simulink model "point_cloud_fusion_node"  (R2016b)
settings: Solver=FixedStepAuto  StartTime=0.0  StopTime=10.0  RelTol=1e-3
model workspace (MAT data in the model file):
  Logfile_Data_Object = [3707764736; 2; 1; 1; 1; 4]
  Logfile_Path = 'C:\Users\takum\MATLAB\Projects\Autoware.Auto\ros2bag\lidars_point_raw\lidars_point_raw_0.db3'
  Logfile_Playback_Duration = nan
  Logfile_Playback_Offset = nan
  SL_ROS_VariableLengthArrays_MaxSizes.CommonInfo.ArrayTruncateAction = 'EmitWarning'
  SL_ROS_VariableLengthArrays_MaxSizes.MsgTypeMap = containers.Map
  SL_ROS_VariableLengthArrays_MaxSizes.MsgTypeMap.serialization.keys = {'sensor_msgs/PointCloud2'}
  SL_ROS_VariableLengthArrays_MaxSizes.MsgTypeMap.serialization.values{1}(1).PropertyName = 'data'
  SL_ROS_VariableLengthArrays_MaxSizes.MsgTypeMap.serialization.values{1}(1).DataType = 'uint8'
  SL_ROS_VariableLengthArrays_MaxSizes.MsgTypeMap.serialization.values{1}(1).MaxLength = 130752
  SL_ROS_VariableLengthArrays_MaxSizes.MsgTypeMap.serialization.values{1}(2).PropertyName = 'fields'
  SL_ROS_VariableLengthArrays_MaxSizes.MsgTypeMap.serialization.values{1}(2).DataType = 'sensor_msgs/PointField'
  SL_ROS_VariableLengthArrays_MaxSizes.MsgTypeMap.serialization.values{1}(2).MaxLength = 16
  SL_ROS_VariableLengthArrays_MaxSizes.MsgTypeMap.serialization.uniformity = 0
  SL_ROS_VariableLengthArrays_MaxSizes.MsgTypeMap.serialization.keyType = 'char'
  SL_ROS_VariableLengthArrays_MaxSizes.MsgTypeMap.serialization.valueType = 'any'
undefined symbols (not defined in the file): data, header, height, row_step, width
libraries: simulink x4
settings Model: Creator=takum  LastModifiedBy=takum
settings DataIOCC: ReturnWorkspaceOutputs=on
settings OptimizationCC: EnhancedBackFolding=on  PassReuseOutputArgsAs=Individual arguments  MaxStackSize=64
settings DebuggingCC: ParameterTunabilityLossMsg=error
settings SFSimCC: SimUseLocalCustomCode=on
settings RTWCC: SystemTargetFile=ert.tlc  HardwareBoard=Robot Operating System 2 (ROS 2)  TLCOptions=-aInlineSetEventsForThisBaseRateFcn=TLC_FALSE -aSuppressMultiTaskScheduler=TLC_FALSE -aRateBasedStepFcn=1  TemplateMakefile=ert_default_tmf  Description=Embedded Coder  RTWUseLocalCustomCode=on  Toolchain=Colcon Tools  TargetLang=C++
settings CodeAppCC: ForceParamTrailComments=on  IgnoreCustomStorageClasses=off  OperatorAnnotations=on  SimulinkDataObjDesc=on  SFDataObjDesc=on  InsertBlockDesc=on
settings ERTTargetCC: MultiwordLength=256  MultiInstanceERTCode=on  CodeInterfacePackaging=C++ class  RootIOFormat=Structure reference

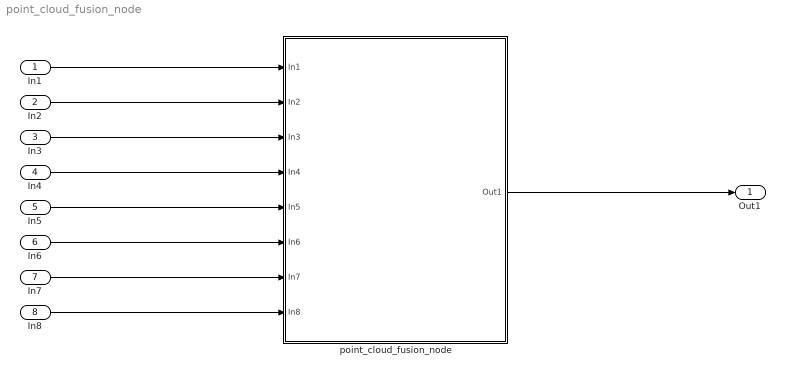
== system point_cloud_fusion_node ==
  In1 : Inport  OutDataTypeStr=Bus: SL_Bus_sensor_msgs_PointCloud2
  In2 : Inport  Port=2  OutDataTypeStr=Bus: SL_Bus_sensor_msgs_PointCloud2
  In3 : Inport  Port=3  OutDataTypeStr=Bus: SL_Bus_sensor_msgs_PointCloud2
  In4 : Inport  Port=4  OutDataTypeStr=Bus: SL_Bus_sensor_msgs_PointCloud2
  In5 : Inport  Port=5  OutDataTypeStr=Bus: SL_Bus_sensor_msgs_PointCloud2
  In6 : Inport  Port=6  OutDataTypeStr=Bus: SL_Bus_sensor_msgs_PointCloud2
  In7 : Inport  Port=7  OutDataTypeStr=Bus: SL_Bus_sensor_msgs_PointCloud2
  In8 : Inport  Port=8  OutDataTypeStr=Bus: SL_Bus_sensor_msgs_PointCloud2
  point_cloud_fusion_node : Subsystem  TreatAsAtomicUnit=on
  Out1 : Outport  OutDataTypeStr=Bus: SL_Bus_sensor_msgs_PointCloud2
  wires:
  point_cloud_fusion_node/1(Out1) -> Out1/1
  In1/1 -> point_cloud_fusion_node/1(In1)
  In2/1 -> point_cloud_fusion_node/2(In2)
  In3/1 -> point_cloud_fusion_node/3(In3)
  In4/1 -> point_cloud_fusion_node/4(In4)
  In5/1 -> point_cloud_fusion_node/5(In5)
  In6/1 -> point_cloud_fusion_node/6(In6)
  In7/1 -> point_cloud_fusion_node/7(In7)
  In8/1 -> point_cloud_fusion_node/8(In8)

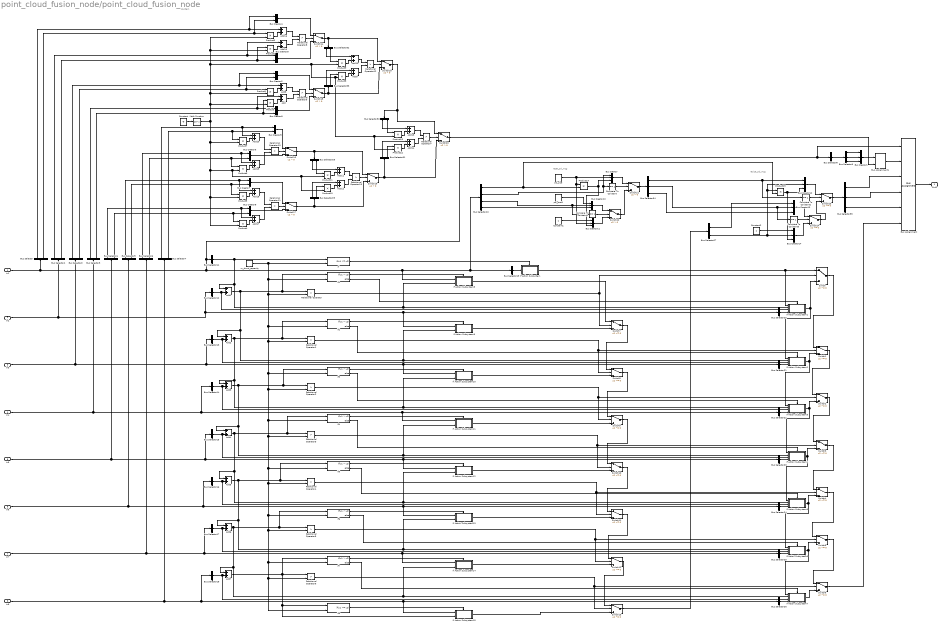
== system point_cloud_fusion_node/point_cloud_fusion_node ==
  note: Subsystem
  note: reset_pcl_msg
  note: resize_pcl_msg
  In1 : Inport
  In2 : Inport  Port=2
  In3 : Inport  Port=3
  In4 : Inport  Port=4
  In5 : Inport  Port=5
  In6 : Inport  Port=6
  In7 : Inport  Port=7
  In8 : Inport  Port=8
  Add{,1..20} (21 alike) : Sum
  Bus Assignment : BusAssignment  AssignedSignals=header,height,width,row_step,data
  Bus Assignment1 : BusAssignment  AssignedSignals=stamp
  Bus Creator{,1,10..14} (7 alike) : BusCreator  Inputs=3
  Bus Creator{2..9} (8 alike) : BusCreator  Inputs=2
  Bus Selector{,1..7} (8 alike) : BusSelector  OutputSignals=header.stamp.sec,header.stamp.nanosec
  Bus Selector10 : BusSelector  OutputSignals=point_step,height,width,row_step
  Bus Selector{11..18} (8 alike) : BusSelector  OutputSignals=width
  Bus Selector{19..26} (8 alike) : BusSelector  OutputSignals=data
  Bus Selector27 : BusSelector  OutputSignals=height,width
  Bus Selector{28..33} (6 alike) : BusSelector  OutputSignals=sec,nanosec
  Bus Selector34 : BusSelector  OutputSignals=height,width,row_step
  Bus Selector35 : BusSelector  OutputSignals=height,width,row_step
  Bus Selector8 : BusSelector  OutputSignals=header
  Bus Selector9 : BusSelector  OutputSignals=stamp,frame_id,frame_id_SL_Info
  Compare To Constant{,1..3} (4 alike) : simulink/Logic and Bit Operations/Compare To Constant  relop===  const=1  OutDataTypeStr=boolean
  Constant : Constant  Value=-9
  Constant1 : Constant
  Constant2 : Constant
  If : If  NumInputs=2  IfExpression=u1 <= u2  ShowElse=off
  If Action Subsystem : Subsystem  TreatAsAtomicUnit=on
  If Action Subsystem1 : Subsystem  TreatAsAtomicUnit=on
  If Action Subsystem10 : Subsystem  TreatAsAtomicUnit=on
  If Action Subsystem11 : Subsystem  TreatAsAtomicUnit=on
  If Action Subsystem12 : Subsystem  TreatAsAtomicUnit=on
  If Action Subsystem13 : Subsystem  TreatAsAtomicUnit=on
  If Action Subsystem14 : Subsystem  TreatAsAtomicUnit=on
  If Action Subsystem15 : Subsystem  TreatAsAtomicUnit=on
  If Action Subsystem2 : Subsystem  TreatAsAtomicUnit=on
  If Action Subsystem3 : Subsystem  TreatAsAtomicUnit=on
  If Action Subsystem4 : Subsystem  TreatAsAtomicUnit=on
  If Action Subsystem5 : Subsystem  TreatAsAtomicUnit=on
  If Action Subsystem6 : Subsystem  TreatAsAtomicUnit=on
  If Action Subsystem7 : Subsystem  TreatAsAtomicUnit=on
  If Action Subsystem8 : Subsystem  TreatAsAtomicUnit=on
  If Action Subsystem9 : Subsystem  TreatAsAtomicUnit=on
  If{1..7} (7 alike) : If  NumInputs=2  IfExpression=u1 > u2
  If8 : If  NumInputs=2  IfExpression=u1 <= u2  ShowElse=off
  Math Function : Math  Operator=10^u  SaturateOnIntegerOverflow=on
  Product{,1..15} (16 alike) : Product
  Relational Operator{,1..13} (14 alike) : RelationalOperator  Operator=>  OutDataTypeStr=boolean  RndMeth=Simplest
  Switch{,1..13,23..24} (16 alike) : Switch  Criteria=u2 ~= 0
  Switch{14..22} (9 alike) : Switch  Criteria=u2 > Threshold
  m_cloud_capacity : Constant  Value=55000  OutDataTypeStr=uint32
  pcl_size : Constant  Value=55000
  pcl_size1 : Constant  Value=55000
  Out1 : Outport
  wires:
  In1/1 -> Bus Selector/1, Bus Selector11/1, Bus Assignment/1, Bus Selector8/1, Bus Selector19/1, Bus Selector10/1, If Action Subsystem8/1(In1)
  Relational Operator12/1 -> Switch18/2
  If4/1 -> If Action Subsystem11/Action
  Compare To Constant1/1 -> Switch22/2
  Bus Creator/1 -> Switch21/1
  If Action Subsystem9/1(Out1) -> Switch7/3
  Bus Selector1/1 -> Add15/1, Bus Creator3/1  "<sec>"
  If Action Subsystem1/1(msgs) -> Switch/3, If Action Subsystem2/1(In1)
  In8/1 -> Bus Selector7/1, If Action Subsystem15/1(In1), Bus Selector26/1, Bus Selector18/1
  Relational Operator11/1 -> Switch17/2
  Bus Selector34/3 -> Bus Creator13/3  "<row_step>"
  If5/1 -> If Action Subsystem12/Action
  If7/2 -> If Action Subsystem7/Action
  Bus Selector1/2 -> Product2/1, Bus Creator3/2  "<nanosec>"
  Add15/1 -> Relational Operator8/2
  Add20/1 -> Relational Operator10/1
  Bus Selector33/1 -> Add9/1  "<sec>"
  Switch10/1 -> Switch11/1
  Compare To Constant/1 -> Switch21/2
  If Action Subsystem2/1(msgs) -> If Action Subsystem3/1(In1), Switch1/3
  Bus Selector10/1 -> Product15/2, Product14/2  "<point_step>"
  Bus Selector19/1 -> If Action Subsystem/1(pc_in)  "<data>"
  In3/1 -> Bus Selector2/1, Bus Selector13/1, Bus Selector21/1, If Action Subsystem10/1(In1)
  Product4/1 -> Add17/2
  Switch21/1 -> Bus Selector34/1
  Bus Selector6/1 -> Add19/1, Bus Creator6/1  "<sec>"
  Constant2/1 -> Bus Creator14/1  "height"
  Relational Operator6/1 -> Switch13/2, Switch6/2
  Product3/1 -> Add16/2
  If Action Subsystem7/1(msgs) -> Switch6/3
  Product14/1 -> Bus Creator11/3, Bus Creator/3  "row_step"
  Switch9/1 -> Switch10/1
  If1/1 -> If Action Subsystem8/Action
  Compare To Constant3/1 -> Switch24/2
  Bus Assignment/1 -> Out1/1
  Product15/1 -> Bus Creator12/3, Bus Creator14/3  "row_step"
  Bus Selector14/1 -> If Action Subsystem3/3(In3), Add3/2  "<width>"
  Bus Creator10/1 -> Switch22/1
  Compare To Constant2/1 -> Switch23/2
  Switch23/1 -> Bus Selector35/1
  If Action Subsystem12/1(Out1) -> Switch10/3
  Product2/1 -> Add15/2
  Bus Selector2/1 -> Bus Creator2/1, Add8/1  "<sec>"
  Bus Creator6/1 -> Switch16/3
  Relational Operator13/1 -> Switch19/2
  Bus Selector7/1 -> Add20/1, Bus Creator5/1  "<sec>"
  Relational Operator7/1 -> Switch20/2
  If3/1 -> If Action Subsystem10/Action
  Relational Operator8/1 -> Switch14/2
  Bus Creator12/1 -> Switch23/1
  Bus Selector21/1 -> If Action Subsystem2/4(pc_in)  "<data>"
  Switch4/1 -> Switch5/1
  Bus Selector24/1 -> If Action Subsystem5/4(pc_in)  "<data>"
  Switch2/1 -> Switch3/1
  Bus Selector27/2 -> Bus Creator12/2, Product15/1, Bus Creator14/2  "<width>"
  Bus Selector31/2 -> Product12/1  "<nanosec>"
  Bus Selector35/1 -> Bus Assignment/3  "<height>"
  If Action Subsystem3/1(msgs) -> If Action Subsystem4/1(In1), Switch2/3
  Switch14/1 -> Switch18/1, Bus Selector32/1
  Bus Selector23/1 -> If Action Subsystem4/4(pc_in)  "<data>"
  If6/2 -> If Action Subsystem6/Action
  If Action Subsystem11/1(Out1) -> Switch9/3
  Product6/1 -> Add19/2
  Product7/1 -> Add20/2
  Add3/1 -> If3/1, Relational Operator2/1, Add4/1, If Action Subsystem4/2(<width>), If Action Subsystem11/2(In2)
  Add2/1 -> If2/1, Relational Operator1/1, If Action Subsystem10/2(In2), If Action Subsystem3/2(<width>), Add3/1
  Bus Assignment1/1 -> Bus Assignment/2
  Relational Operator9/1 -> Switch15/2
  Switch3/1 -> Switch4/1
  If4/2 -> If Action Subsystem4/Action
  Add13/1 -> Relational Operator7/1
  Bus Selector30/2 -> Product13/1  "<nanosec>"
  Bus Selector28/1 -> Add11/1  "<sec>"
  Relational Operator10/1 -> Switch16/2
  Product/1 -> Add/2
  Bus Selector10/3 -> Compare To Constant1/1, Bus Creator10/2  "<width>"
  Bus Selector7/2 -> Bus Creator5/2, Product7/1  "<nanosec>"
  Bus Creator13/1 -> Switch24/1
  Bus Selector34/1 -> Compare To Constant2/1, Bus Creator12/1  "<height>"
  Switch/1 -> Switch1/1
  If2/2 -> If Action Subsystem2/Action
  If3/2 -> If Action Subsystem3/Action
  Bus Selector10/4 -> Bus Creator10/3  "<row_step>"
  Add16/1 -> Relational Operator8/1
  Add1/1 -> If Action Subsystem9/2(In2), If Action Subsystem2/2(<width>), Add2/1, Relational Operator/1, If1/1
  Bus Selector9/1 -> Bus Creator1/1  "<stamp>"
  Bus Selector5/2 -> Bus Creator7/2, Product5/1  "<nanosec>"
  In6/1 -> Bus Selector5/1, Bus Selector24/1, If Action Subsystem13/1(In1), Bus Selector16/1
  Add/1 -> Relational Operator9/2
  Switch12/1 -> Switch13/1
  Math Function/1 -> Product4/2, Product5/2, Product10/2, Product11/2, Product6/2, Product7/2, Product2/2, Product3/2, Product13/2, Product12/2, Product8/2, Product9/2, Product1/2, Product/2
  If Action Subsystem/1(msgs) -> If Action Subsystem1/1(In1), Switch/1
  Bus Selector35/2 -> Bus Assignment/4  "<width>"
  Bus Selector10/2 -> Bus Creator/1, Compare To Constant/1  "<height>"
  Bus Selector18/1 -> If Action Subsystem7/3(In3), Add7/2  "<width>"
  pcl_size/1 -> Bus Creator/2, Bus Creator11/2, Product14/1  "width"
  Bus Selector29/1 -> Add12/1  "<sec>"
  Bus Selector6/2 -> Bus Creator6/2, Product6/1  "<nanosec>"
  Bus Creator11/1 -> Switch22/3
  Bus Selector9/2 -> Bus Creator1/2  "<frame_id>"
  Product8/1 -> Add9/2
  Bus Selector25/1 -> If Action Subsystem6/4(pc_in)  "<data>"
  If Action Subsystem15/1(Out1) -> Switch13/3
  If Action Subsystem13/1(Out1) -> Switch11/3
  Switch22/1 -> Switch21/3
  Switch17/1 -> Switch19/3, Bus Selector29/1
  Bus Selector34/2 -> Compare To Constant3/1, Bus Creator13/2  "<width>"
  Bus Creator9/1 -> Switch15/3
  If Action Subsystem8/1(Out1) -> Switch7/1
  Relational Operator3/1 -> Switch10/2, Switch3/2
  Switch18/1 -> Bus Selector30/1, Switch20/1
  Add18/1 -> Relational Operator11/1
  In7/1 -> Bus Selector6/1, If Action Subsystem14/1(In1), Bus Selector25/1, Bus Selector17/1
  Relational Operator2/1 -> Switch2/2, Switch9/2
  Add14/1 -> Relational Operator7/2
  Product5/1 -> Add18/2
  Add17/1 -> Relational Operator11/2
  Bus Selector17/1 -> If Action Subsystem6/3(In3), Add6/2  "<width>"
  If1/2 -> If Action Subsystem1/Action
  Product12/1 -> Add14/2
  Switch19/1 -> Bus Selector31/1, Switch20/3
  If2/1 -> If Action Subsystem9/Action
  Bus Creator2/1 -> Switch15/1
  Add8/1 -> Relational Operator9/1
  Add9/1 -> Relational Operator12/2
  Bus Creator14/1 -> Switch24/3
  If8/1 -> If Action Subsystem15/Action
  In4/1 -> Bus Selector3/1, If Action Subsystem11/1(In1), Bus Selector22/1, Bus Selector14/1
  Bus Creator1/1 -> Bus Assignment1/1
  Product10/1 -> Add12/2
  Add6/1 -> If Action Subsystem14/2(In2), If Action Subsystem7/2(<width>), Add7/1, If6/1, Relational Operator5/1
  Switch1/1 -> Switch2/1
  Switch6/1 -> Bus Assignment/6  "data"
  Add5/1 -> If5/1, Relational Operator4/1, If Action Subsystem13/2(In2), If Action Subsystem6/2(<width>), Add6/1
  If Action Subsystem4/1(msgs) -> If Action Subsystem5/1(In1), Switch3/3
  Product1/1 -> Add8/2
  Add11/1 -> Relational Operator13/1
  Constant1/1 -> Bus Creator11/1  "height"
  If Action Subsystem10/1(Out1) -> Switch8/3
  If Action Subsystem5/1(msgs) -> If Action Subsystem6/1(In1), Switch4/3
  If7/1 -> If Action Subsystem14/Action
  Bus Selector12/1 -> If Action Subsystem1/3(In3), Add1/2  "<width>"
  Add12/1 -> Relational Operator13/2
  If5/2 -> If Action Subsystem5/Action
  Constant/1 -> Math Function/1
  Switch24/1 -> Switch23/3
  Bus Creator8/1 -> Switch17/3
  Bus Selector15/1 -> If Action Subsystem4/3(In3), Add4/2  "<width>"
  Bus Creator7/1 -> Switch17/1
  Switch5/1 -> Switch6/1
  Switch20/1 -> Bus Assignment1/2  "header.stamp"
  Bus Selector9/3 -> Bus Creator1/3  "<frame_id_SL_Info>"
  Bus Selector33/2 -> Product8/1  "<nanosec>"
  Bus Selector/1 -> Add16/1, Bus Creator4/1  "<sec>"
  Bus Selector20/1 -> If Action Subsystem1/4(pc_in)  "<data>"
  Relational Operator5/1 -> Switch12/2, Switch5/2
  Bus Selector29/2 -> Product10/1  "<nanosec>"
  Product13/1 -> Add13/2
  Bus Creator5/1 -> Switch16/1
  Bus Selector8/1 -> Bus Selector9/1  "<header>"
  Bus Selector22/1 -> If Action Subsystem3/4(pc_in)  "<data>"
  m_cloud_capacity/1 -> Relational Operator3/2, Relational Operator4/2, If8/2, Relational Operator6/2, If7/2, Relational Operator5/2, If6/2, If5/2, If4/2, Relational Operator2/2, If3/2, Relational Operator1/2, If2/2, Relational Operator/2, If1/2, If/2
  Add10/1 -> Relational Operator12/1
  Add7/1 -> If8/1, If Action Subsystem15/2(In2), If7/1, Relational Operator6/1
  Bus Selector26/1 -> If Action Subsystem7/4(pc_in)  "<data>"
  Bus Selector/2 -> Product3/1, Bus Creator4/2  "<nanosec>"
  Bus Selector16/1 -> If Action Subsystem5/3(In3), Add5/2  "<width>"
  If Action Subsystem14/1(Out1) -> Switch12/3
  Relational Operator1/1 -> Switch8/2, Switch1/2
  If6/1 -> If Action Subsystem13/Action
  Product9/1 -> Add10/2
  Switch13/1 -> Bus Selector27/1
  Bus Selector31/1 -> Add14/1  "<sec>"
  Bus Selector32/1 -> Add10/1  "<sec>"
  Bus Selector3/2 -> Bus Creator9/2, Product/1  "<nanosec>"
  Bus Creator3/1 -> Switch14/3
  Bus Selector32/2 -> Product9/1  "<nanosec>"
  Bus Selector11/1 -> If Action Subsystem1/2(<width>), If Action Subsystem8/2(In2), Add1/1, If/1  "<width>"
  Relational Operator4/1 -> Switch11/2, Switch4/2
  Switch8/1 -> Switch9/1
  Bus Selector4/1 -> Bus Creator8/1, Add17/1  "<sec>"
  If/1 -> If Action Subsystem/Action
  If Action Subsystem6/1(msgs) -> If Action Subsystem7/1(In1), Switch5/3
  Bus Selector2/2 -> Bus Creator2/2, Product1/1  "<nanosec>"
  pcl_size1/1 -> Bus Creator10/1  "height"
  Bus Selector30/1 -> Add13/1  "<sec>"
  Bus Selector5/1 -> Bus Creator7/1, Add18/1  "<sec>"
  Switch7/1 -> Switch8/1
  Switch15/1 -> Bus Selector33/1, Switch18/3
  Product11/1 -> Add11/2
  Bus Selector13/1 -> If Action Subsystem2/3(In3), Add2/2  "<width>"
  Add19/1 -> Relational Operator10/2
  Bus Selector4/2 -> Bus Creator8/2, Product4/1  "<nanosec>"
  Relational Operator/1 -> Switch/2, Switch7/2
  Add4/1 -> If Action Subsystem12/2(In2), If Action Subsystem5/2(<width>), Add5/1, If4/1, Relational Operator3/1
  Bus Creator4/1 -> Switch14/1
  In2/1 -> Bus Selector1/1, If Action Subsystem9/1(In1), Bus Selector20/1, Bus Selector12/1
  Bus Selector35/3 -> Bus Assignment/5  "<row_step>"
  Switch11/1 -> Switch12/1
  Bus Selector3/1 -> Bus Creator9/1, Add/1  "<sec>"
  Bus Selector28/2 -> Product11/1  "<nanosec>"
  Bus Selector27/1 -> Bus Creator13/1  "<height>"
  In5/1 -> Bus Selector4/1, Bus Selector23/1, If Action Subsystem12/1(In1), Bus Selector15/1
  Switch16/1 -> Switch19/1, Bus Selector28/1

== system point_cloud_fusion_node/point_cloud_fusion_node/If Action Subsystem ==
  pc_in : Inport
  Action Port : ActionPort  ActionType=then
  msgs : Outport
  wires:
  pc_in/1 -> msgs/1

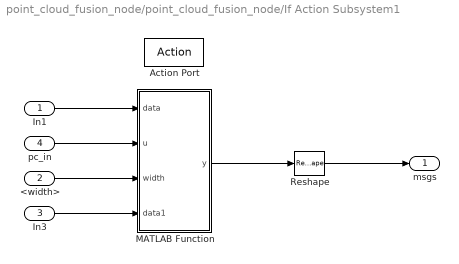
== system point_cloud_fusion_node/point_cloud_fusion_node/If Action Subsystem1 ==
  In1 : Inport
  <width> : Inport  Port=2
  In3 : Inport  Port=3
  pc_in : Inport  Port=4
  Action Port : ActionPort  ActionType=else
  MATLAB Function : MATLAB Function  TreatAsAtomicUnit=on
  Reshape : Reshape
  msgs : Outport
  wires:
  pc_in/1 -> MATLAB Function/2(u)
  MATLAB Function/1(y) -> Reshape/1
  In1/1 -> MATLAB Function/1(data)
  <width>/1 -> MATLAB Function/3(width)
  In3/1 -> MATLAB Function/4(data1)
  Reshape/1 -> msgs/1

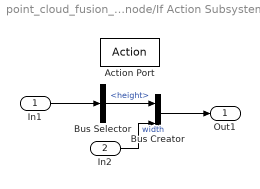
== system point_cloud_fusion_node/point_cloud_fusion_node/If Action Subsystem10 ==
  In1 : Inport
  In2 : Inport  Port=2
  Action Port : ActionPort  ActionType=then
  Bus Creator : BusCreator  Inputs=2
  Bus Selector : BusSelector  OutputSignals=height
  Out1 : Outport
  wires:
  In1/1 -> Bus Selector/1
  Bus Selector/1 -> Bus Creator/1  "<height>"
  Bus Creator/1 -> Out1/1
  In2/1 -> Bus Creator/2  "width"

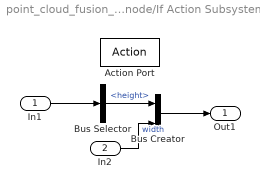
== system point_cloud_fusion_node/point_cloud_fusion_node/If Action Subsystem11 ==
  In1 : Inport
  In2 : Inport  Port=2
  Action Port : ActionPort  ActionType=then
  Bus Creator : BusCreator  Inputs=2
  Bus Selector : BusSelector  OutputSignals=height
  Out1 : Outport
  wires:
  In1/1 -> Bus Selector/1
  Bus Selector/1 -> Bus Creator/1  "<height>"
  Bus Creator/1 -> Out1/1
  In2/1 -> Bus Creator/2  "width"

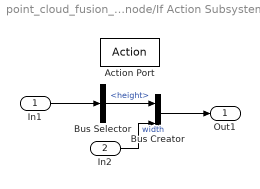
== system point_cloud_fusion_node/point_cloud_fusion_node/If Action Subsystem12 ==
  In1 : Inport
  In2 : Inport  Port=2
  Action Port : ActionPort  ActionType=then
  Bus Creator : BusCreator  Inputs=2
  Bus Selector : BusSelector  OutputSignals=height
  Out1 : Outport
  wires:
  In1/1 -> Bus Selector/1
  Bus Selector/1 -> Bus Creator/1  "<height>"
  Bus Creator/1 -> Out1/1
  In2/1 -> Bus Creator/2  "width"

== system point_cloud_fusion_node/point_cloud_fusion_node/If Action Subsystem13 ==
  In1 : Inport
  In2 : Inport  Port=2
  Action Port : ActionPort  ActionType=then
  Bus Creator1 : BusCreator  Inputs=2
  Bus Selector1 : BusSelector  OutputSignals=height
  Out1 : Outport
  wires:
  Bus Creator1/1 -> Out1/1
  In2/1 -> Bus Creator1/2  "width"
  Bus Selector1/1 -> Bus Creator1/1  "<height>"
  In1/1 -> Bus Selector1/1

== system point_cloud_fusion_node/point_cloud_fusion_node/If Action Subsystem14 ==
  In1 : Inport
  In2 : Inport  Port=2
  Action Port : ActionPort  ActionType=then
  Bus Creator : BusCreator  Inputs=2
  Bus Selector : BusSelector  OutputSignals=height
  Out1 : Outport
  wires:
  In1/1 -> Bus Selector/1
  Bus Selector/1 -> Bus Creator/1  "<height>"
  Bus Creator/1 -> Out1/1
  In2/1 -> Bus Creator/2  "width"

== system point_cloud_fusion_node/point_cloud_fusion_node/If Action Subsystem15 ==
  In1 : Inport
  In2 : Inport  Port=2
  Action Port : ActionPort  ActionType=then
  Bus Creator : BusCreator  Inputs=2
  Bus Selector : BusSelector  OutputSignals=height
  Out1 : Outport
  wires:
  In1/1 -> Bus Selector/1
  Bus Selector/1 -> Bus Creator/1  "<height>"
  Bus Creator/1 -> Out1/1
  In2/1 -> Bus Creator/2  "width"

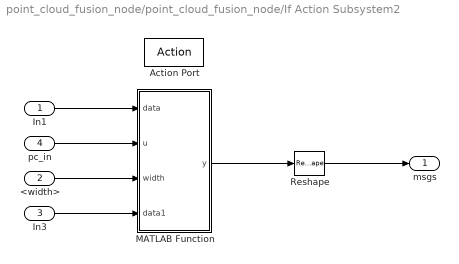
== system point_cloud_fusion_node/point_cloud_fusion_node/If Action Subsystem2 ==
  In1 : Inport
  <width> : Inport  Port=2
  In3 : Inport  Port=3
  pc_in : Inport  Port=4
  Action Port : ActionPort  ActionType=else
  MATLAB Function : MATLAB Function  TreatAsAtomicUnit=on
  Reshape : Reshape
  msgs : Outport
  wires:
  pc_in/1 -> MATLAB Function/2(u)
  MATLAB Function/1(y) -> Reshape/1
  In1/1 -> MATLAB Function/1(data)
  <width>/1 -> MATLAB Function/3(width)
  In3/1 -> MATLAB Function/4(data1)
  Reshape/1 -> msgs/1

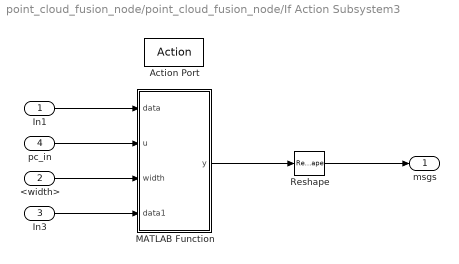
== system point_cloud_fusion_node/point_cloud_fusion_node/If Action Subsystem3 ==
  In1 : Inport
  <width> : Inport  Port=2
  In3 : Inport  Port=3
  pc_in : Inport  Port=4
  Action Port : ActionPort  ActionType=else
  MATLAB Function : MATLAB Function  TreatAsAtomicUnit=on
  Reshape : Reshape
  msgs : Outport
  wires:
  pc_in/1 -> MATLAB Function/2(u)
  MATLAB Function/1(y) -> Reshape/1
  In1/1 -> MATLAB Function/1(data)
  <width>/1 -> MATLAB Function/3(width)
  In3/1 -> MATLAB Function/4(data1)
  Reshape/1 -> msgs/1

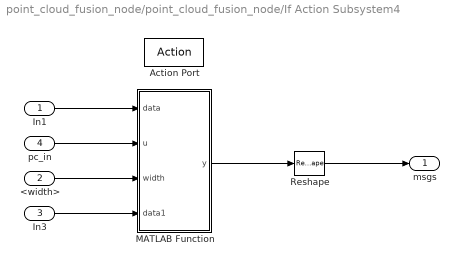
== system point_cloud_fusion_node/point_cloud_fusion_node/If Action Subsystem4 ==
  In1 : Inport
  <width> : Inport  Port=2
  In3 : Inport  Port=3
  pc_in : Inport  Port=4
  Action Port : ActionPort  ActionType=else
  MATLAB Function : MATLAB Function  TreatAsAtomicUnit=on
  Reshape : Reshape
  msgs : Outport
  wires:
  pc_in/1 -> MATLAB Function/2(u)
  MATLAB Function/1(y) -> Reshape/1
  In1/1 -> MATLAB Function/1(data)
  <width>/1 -> MATLAB Function/3(width)
  In3/1 -> MATLAB Function/4(data1)
  Reshape/1 -> msgs/1

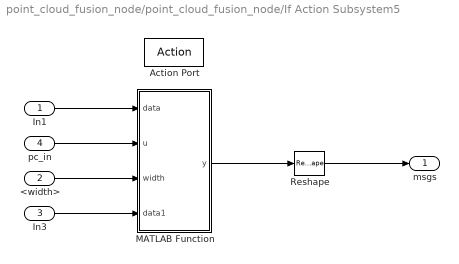
== system point_cloud_fusion_node/point_cloud_fusion_node/If Action Subsystem5 ==
  In1 : Inport
  <width> : Inport  Port=2
  In3 : Inport  Port=3
  pc_in : Inport  Port=4
  Action Port : ActionPort  ActionType=else
  MATLAB Function : MATLAB Function  TreatAsAtomicUnit=on
  Reshape : Reshape
  msgs : Outport
  wires:
  pc_in/1 -> MATLAB Function/2(u)
  MATLAB Function/1(y) -> Reshape/1
  In1/1 -> MATLAB Function/1(data)
  <width>/1 -> MATLAB Function/3(width)
  In3/1 -> MATLAB Function/4(data1)
  Reshape/1 -> msgs/1

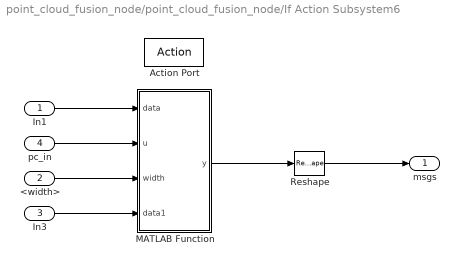
== system point_cloud_fusion_node/point_cloud_fusion_node/If Action Subsystem6 ==
  In1 : Inport
  <width> : Inport  Port=2
  In3 : Inport  Port=3
  pc_in : Inport  Port=4
  Action Port : ActionPort  ActionType=else
  MATLAB Function : MATLAB Function  TreatAsAtomicUnit=on
  Reshape : Reshape
  msgs : Outport
  wires:
  pc_in/1 -> MATLAB Function/2(u)
  MATLAB Function/1(y) -> Reshape/1
  In1/1 -> MATLAB Function/1(data)
  <width>/1 -> MATLAB Function/3(width)
  In3/1 -> MATLAB Function/4(data1)
  Reshape/1 -> msgs/1

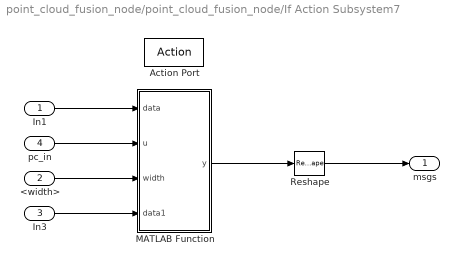
== system point_cloud_fusion_node/point_cloud_fusion_node/If Action Subsystem7 ==
  In1 : Inport
  <width> : Inport  Port=2
  In3 : Inport  Port=3
  pc_in : Inport  Port=4
  Action Port : ActionPort  ActionType=else
  MATLAB Function : MATLAB Function  TreatAsAtomicUnit=on
  Reshape : Reshape
  msgs : Outport
  wires:
  pc_in/1 -> MATLAB Function/2(u)
  MATLAB Function/1(y) -> Reshape/1
  In1/1 -> MATLAB Function/1(data)
  <width>/1 -> MATLAB Function/3(width)
  In3/1 -> MATLAB Function/4(data1)
  Reshape/1 -> msgs/1

== system point_cloud_fusion_node/point_cloud_fusion_node/If Action Subsystem8 ==
  In1 : Inport
  In2 : Inport  Port=2
  Action Port : ActionPort  ActionType=then
  Bus Creator : BusCreator  Inputs=2
  Bus Selector : BusSelector  OutputSignals=height
  Out1 : Outport
  wires:
  In1/1 -> Bus Selector/1
  Bus Selector/1 -> Bus Creator/1  "<height>"
  Bus Creator/1 -> Out1/1
  In2/1 -> Bus Creator/2  "width"

== system point_cloud_fusion_node/point_cloud_fusion_node/If Action Subsystem9 ==
  In1 : Inport
  In2 : Inport  Port=2
  Action Port : ActionPort  ActionType=then
  Bus Creator : BusCreator  Inputs=2
  Bus Selector : BusSelector  OutputSignals=height
  Out1 : Outport
  wires:
  In1/1 -> Bus Selector/1
  Bus Selector/1 -> Bus Creator/1  "<height>"
  Bus Creator/1 -> Out1/1
  In2/1 -> Bus Creator/2  "width"

== matlab function point_cloud_fusion_node/If Action Subsystem2/MATLAB Function ==
  data: data input; u input; y output; width input; data1 input
function y = fcn(data, u, width, data1)
s=width+1;
f=width+data1;
data(s:f)=u(1:data1);
y=data;

== matlab function point_cloud_fusion_node/If Action Subsystem1/MATLAB Function ==
  data: data input; u input; y output; width input; data1 input
function y = fcn(data, u, width, data1)
s=width+1;
f=width+data1;
data(s:f)=u(1:data1);
y=data;

== matlab function point_cloud_fusion_node/If Action Subsystem3/MATLAB Function ==
  data: data input; u input; y output; width input; data1 input
function y = fcn(data, u, width, data1)
s=width+1;
f=width+data1;
data(s:f)=u(1:data1);
y=data;

== matlab function point_cloud_fusion_node/If Action Subsystem4/MATLAB Function ==
  data: data input; u input; y output; width input; data1 input
function y = fcn(data, u, width, data1)
s=width+1;
f=width+data1;
data(s:f)=u(1:data1);
y=data;

== matlab function point_cloud_fusion_node/If Action Subsystem5/MATLAB Function ==
  data: data input; u input; y output; width input; data1 input
function y = fcn(data, u, width, data1)
s=width+1;
f=width+data1;
data(s:f)=u(1:data1);
y=data;

== matlab function point_cloud_fusion_node/If Action Subsystem6/MATLAB Function ==
  data: data input; u input; y output; width input; data1 input
function y = fcn(data, u, width, data1)
s=width+1;
f=width+data1;
data(s:f)=u(1:data1);
y=data;

== matlab function point_cloud_fusion_node/If Action Subsystem7/MATLAB Function ==
  data: data input; u input; y output; width input; data1 input
function y = fcn(data, u, width, data1)
s=width+1;
f=width+data1;
data(s:f)=u(1:data1);
y=data;
